simulink model "FFR_3area_4"  (R2015a)
settings: Solver=ode45  StartTime=0.0  StopTime=30  RelTol=1e-3
values from neighbouring files (symbols this model uses):
  beta = [0.3483 0.3827 0.3692]    [init_FFR_3area.m]    (also in init_FFR_3area_2.m; init_FFR_3area_3.m; init_FFR_3area_4.m; init_FFR_3area_5.m)
  D = 0.015    [init_FFR_1_0.m]    (also in init_FFR_1_1.m; init_FFR_3area.m = [0.015 0.016 0.015]; init_FFR_3area_2.m = [0.015 0.016 0.015]; init_FFR_3area_3.m = [0.015 0.016 0.015])
  H = 0.0833    [init_FFR_1_0.m]    (also in init_FFR_1_1.m; init_FFR_3area.m = [0.1667 0.2017 0.1247] .* 0.5; init_FFR_3area_2.m = [0.1667 0.2017 0.1247] .* 0.5; init_FFR_3area_3.m = [0.1667 0.2017 0.1247] .* 0.5)
  Ki = -0.3    [init_FFR_1_0.m]    (also in init_FFR_1_1.m = -2; init_FFR_3area.m = [-0.3 -0.2 -0.4]; init_FFR_3area_2.m = [-0.3 -0.2 -0.4]; init_FFR_3area_3.m = [-0.3 -0.2 -0.4])
  L = 10000    [init_FFR_3area_4.m]    (also in init_FFR_3area_5.m = 1000; init_FRR_3area_6.m = 1000; init_FRR_4area_1.m = 1000)
  MO_down = sortrows(MO_down, 1)    [allocateProduction.m]    (also in allocation.m; init_FFR_3area_4.m; init_FFR_3area_5.m; init_FRR_3area_6.m)
  MO_up = sortrows(MO_up, 1)    [allocateProduction.m]    (also in allocation.m; init_FFR_3area_4.m; init_FFR_3area_5.m; init_FRR_3area_6.m)
  R = 3    [init_FFR_1_0.m]    (also in init_FFR_1_1.m; init_FFR_3area.m = [3 2.73 2.82]; init_FFR_3area_2.m = [3 2.73 2.82]; init_FFR_3area_3.m = [3 2.73 2.82])
  T_12 = 0.20    (= 0.2)    [allocateProduction.m]    (also in allocation.m; init_FFR_3area.m; init_FFR_3area_2.m; init_FFR_3area_3.m)
  T_13 = 0.25    [allocateProduction.m]    (also in allocation.m; init_FFR_3area.m; init_FFR_3area_2.m; init_FFR_3area_3.m)
  T_21 = 0.20    (= 0.2)    [allocateProduction.m]    (also in allocation.m; init_FFR_3area.m; init_FFR_3area_2.m; init_FFR_3area_3.m)
  T_23 = 0.12    [allocateProduction.m]    (also in allocation.m; init_FFR_3area.m; init_FFR_3area_2.m; init_FFR_3area_3.m)
  T_31 = 0.25    [allocateProduction.m]    (also in allocation.m; init_FFR_3area.m; init_FFR_3area_2.m; init_FFR_3area_3.m)
  T_32 = 0.12    [allocateProduction.m]    (also in allocation.m; init_FFR_3area.m; init_FFR_3area_2.m; init_FFR_3area_3.m)
  T_g = 0.08    [init_FFR_1_0.m]    (also in init_FFR_1_1.m; init_FFR_3area.m = [0.08 0.06 0.07]; init_FFR_3area_2.m = [0.08 0.06 0.07]; init_FFR_3area_3.m = [0.08 0.06 0.07])
  T_t = 0.40    (= 0.4)    [init_FFR_1_0.m]    (also in init_FFR_1_1.m; init_FFR_3area.m = [0.40 0.44 0.30]; init_FFR_3area_2.m = [0.40 0.44 0.30]; init_FFR_3area_3.m = [0.40 0.44 0.30])
libraries: simulink x3, aerolibanimutils x1, dspstat3 x1
settings Model: Creator=tarje  LastModifiedBy=tarje

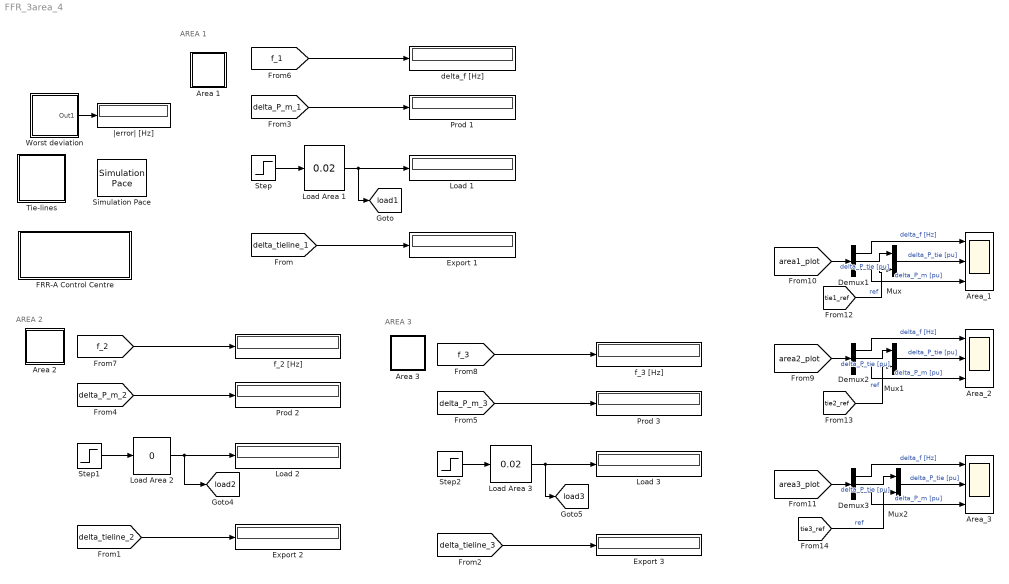
== system FFR_3area_4 ==
  note: AREA 3
  note: AREA 2
  note: AREA 1
  Area 1 : Subsystem
  Area 2 : Subsystem
  Area 3 : Subsystem
  Area_1 : Scope  NumInputPorts=3
      settings: TimeRange=15  YMin=-0.045~-0.015~0.0385  YMax=0.01~0.0175~0.043  SaveName=ScopeData2
  Area_2 : Scope  NumInputPorts=3
      settings: TimeRange=15  YMin=-0.955~-0.2~-0.00045  YMax=-0.855~0.8~0.0007
  Area_3 : Scope  NumInputPorts=3
      settings: TimeRange=15  YMin=-0.965~-0.0575~0.0225  YMax=-0.855~-0.0075~0.0325
  Demux1 : Demux  Outputs=3
  Demux2 : Demux  Outputs=3
  Demux3 : Demux  Outputs=3
  Export 1 : Display
  Export 2 : Display
  Export 3 : Display
  "FRR-A Control Centre " : Subsystem
  Load 1 : Display
  Load 2 : Display
  Load 3 : Display
  Load Area 1 : simulink/Math Operations/Slider Gain  low=-0.2  gain=0.02  high=0.348
  Load Area 2 : simulink/Math Operations/Slider Gain  low=-0.05  gain=0  high=0.348
  Load Area 3 : simulink/Math Operations/Slider Gain  low=-0.05  gain=0.02  high=1
  Mux : Mux  Inputs=2
  Mux1 : Mux  Inputs=2
  Mux2 : Mux  Inputs=2
  Prod 1 : Display
  Prod 2 : Display
  Prod 3 : Display
  Simulation Pace : aerolibanimutils/Simulation Pace  SimulationPace=1  SleepMode=MATLAB Thread  OutputPaceError=off  SampleTime=1/30
      settings: AttributesFormatString=%<SimulationPace> sec/sec
  Step : Step  Time=2  SampleTime=0
  Step1 : Step  Time=2  SampleTime=0
  Step2 : Step  Time=2  SampleTime=0
  Tie-lines : Subsystem
  Worst deviation : Subsystem
  delta_f [Hz] : Display
  f_2 [Hz] : Display
  f_3 [Hz] : Display
  |error| [Hz] : Display
  tag scope: load1=global, load2=global, load3=global
  wires:
  [f_1] -> delta_f [Hz]/1
  [delta_P_m_1] -> Prod 1/1
  Step/1 -> Load Area 1/1
  Load Area 1/1 -> [load1], Load 1/1
  [f_2] -> f_2 [Hz]/1
  [delta_P_m_2] -> Prod 2/1
  Step1/1 -> Load Area 2/1
  Load Area 2/1 -> [load2], Load 2/1
  [f_3] -> f_3 [Hz]/1
  [delta_P_m_3] -> Prod 3/1
  Step2/1 -> Load Area 3/1
  Load Area 3/1 -> [load3], Load 3/1
  [delta_tieline_1] -> Export 1/1
  [delta_tieline_2] -> Export 2/1
  [delta_tieline_3] -> Export 3/1
  Worst deviation/1(Out1) -> |error| [Hz]/1
  [area1_plot] -> Demux1/1
  Demux1/1 -> Area_1/1  "delta_f [Hz]"
  Demux1/2 -> Mux/1  "delta_P_tie [pu]"
  Demux1/3 -> Area_1/3  "delta_P_m [pu]"
  [area2_plot] -> Demux2/1
  Demux2/1 -> Area_2/1  "delta_f [Hz]"
  Demux2/2 -> Mux1/1  "delta_P_tie [pu]"
  Demux2/3 -> Area_2/3  "delta_P_m [pu]"
  [area3_plot] -> Demux3/1
  Demux3/1 -> Area_3/1  "delta_f [Hz]"
  Demux3/2 -> Mux2/1  "delta_P_tie [pu]"
  Demux3/3 -> Area_3/3  "delta_P_m [pu]"
  Mux/1 -> Area_1/2  "delta_P_tie [pu]"
  [tie1_ref] -> Mux/2  "ref"
  [tie2_ref] -> Mux1/2  "ref"
  Mux1/1 -> Area_2/2  "delta_P_tie [pu]"
  Mux2/1 -> Area_3/2  "delta_P_tie [pu]"
  [tie3_ref] -> Mux2/2  "ref"

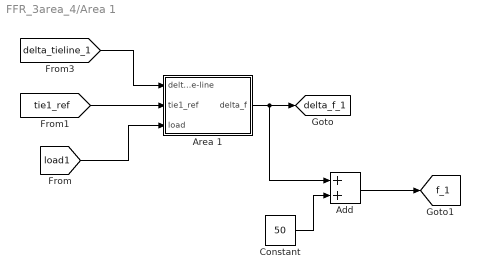
== system FFR_3area_4/Area 1 ==
  Add : Sum
  Area 1 : Subsystem
  Constant : Constant  Value=50
  tag scope: delta_f_1=global, f_1=global
  wires:
  [delta_tieline_1] -> Area 1/1(delta_tie-line)
  Area 1/1(delta_f) -> Add/1, [delta_f_1]
  [load1] -> Area 1/3(load)
  Constant/1 -> Add/2
  Add/1 -> [f_1]
  [tie1_ref] -> Area 1/2(tie1_ref)

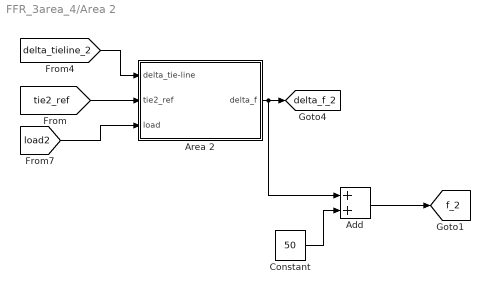
== system FFR_3area_4/Area 2 ==
  Add : Sum
  Area 2 : Subsystem
  Constant : Constant  Value=50
  tag scope: delta_f_2=global, f_2=global
  wires:
  Area 2/1(delta_f) -> Add/1, [delta_f_2]
  [load2] -> Area 2/3(load)
  [delta_tieline_2] -> Area 2/1(delta_tie-line)
  Constant/1 -> Add/2
  Add/1 -> [f_2]
  [tie2_ref] -> Area 2/2(tie2_ref)

== system FFR_3area_4/Area 3 ==
  Add : Sum
  Area 3 : Subsystem
  Constant2 : Constant  Value=50
  tag scope: delta_f_3=global, f_3=global
  wires:
  [load3] -> Area 3/3(load)
  Area 3/1(delta_f) -> Add/1, [delta_f_3]
  [delta_tieline_3] -> Area 3/1(delta_tie-line)
  Add/1 -> [f_3]
  Constant2/1 -> Add/2
  [tie3_ref] -> Area 3/2(tie3_ref)

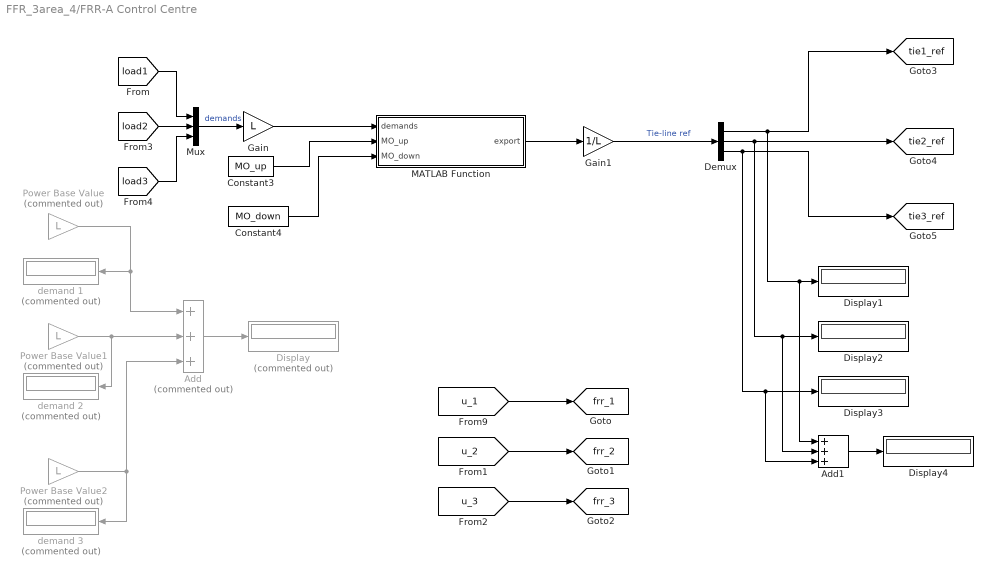
== system FFR_3area_4/FRR-A Control Centre  ==
  Add : Sum  Commented=on  Inputs=+++
  Add1 : Sum  Inputs=3
  Constant3 : Constant  Value=MO_up
  Constant4 : Constant  Value=MO_down
  Demux : Demux  Outputs=3
  Display : Display  Commented=on
  Display{1..4} (4 alike) : Display
  Gain : Gain  Gain=L
  Gain1 : Gain  Gain=1/L
  MATLAB Function : MATLAB Function  TreatAsAtomicUnit=on  SystemSampleTime=2
  Mux : Mux  Inputs=3
  Power Base Value : Gain  Commented=on  Gain=L
  Power Base Value1 : Gain  Commented=on  Gain=L
  Power Base Value2 : Gain  Commented=on  Gain=L
  demand 1 : Display  Commented=on
  demand 2 : Display  Commented=on
  demand 3 : Display  Commented=on
  tag scope: frr_1=global, frr_2=global, frr_3=global, tie1_ref=global, tie2_ref=global, tie3_ref=global
  wires:
  Add/1 -> Display/1
  Power Base Value/1 -> demand 1/1, Add/1
  Power Base Value1/1 -> demand 2/1, Add/2
  Power Base Value2/1 -> demand 3/1, Add/3
  [u_1] -> [frr_1]
  [u_2] -> [frr_2]
  [u_3] -> [frr_3]
  [load2] -> Mux/2
  [load1] -> Mux/1
  [load3] -> Mux/3
  Mux/1 -> Gain/1  "demands"
  Gain1/1 -> Demux/1  "Tie-line ref"
  Constant3/1 -> MATLAB Function/2(MO_up)
  Constant4/1 -> MATLAB Function/3(MO_down)
  Gain/1 -> MATLAB Function/1(demands)
  MATLAB Function/1(export) -> Gain1/1
  Demux/1 -> Add1/1, Display1/1, [tie1_ref]
  Demux/2 -> Add1/2, Display2/1, [tie2_ref]
  Demux/3 -> Add1/3, Display3/1, [tie3_ref]
  Add1/1 -> Display4/1

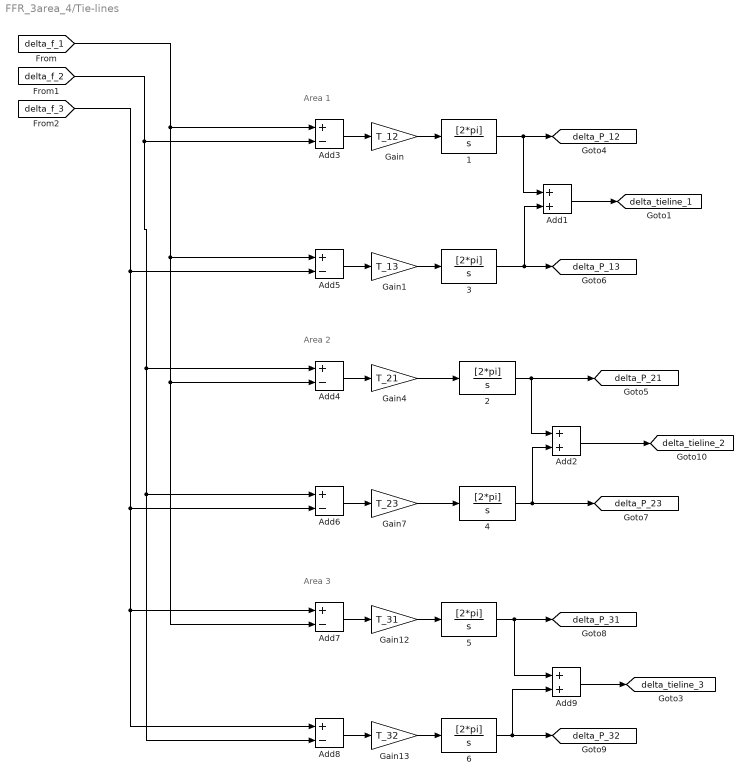
== system FFR_3area_4/Tie-lines ==
  note: Area 3
  note: Area 2
  note: Area 1
   {1..6} (6 alike) : TransferFcn  Numerator=[2*pi]  Denominator=[1 0]
  Add1 : Sum
  Add2 : Sum
  Add{3..8} (6 alike) : Sum  Inputs=+-
  Add9 : Sum
  Gain : Gain  Gain=T_12
  Gain1 : Gain  Gain=T_13
  Gain12 : Gain  Gain=T_31
  Gain13 : Gain  Gain=T_32
  Gain4 : Gain  Gain=T_21
  Gain7 : Gain  Gain=T_23
  tag scope: delta_P_12=global, delta_P_13=global, delta_P_21=global, delta_P_23=global, delta_P_31=global, delta_P_32=global, delta_tieline_1=global, delta_tieline_2=global, delta_tieline_3=global
  wires:
  [delta_f_2] -> Add3/2, Add8/2, Add6/1, Add4/1
  [delta_f_1] -> Add3/1, Add5/1, Add7/2, Add4/2
  [delta_f_3] -> Add5/2, Add8/1, Add7/1, Add6/2
  " 1"/1 -> Add1/1, [delta_P_12]
  Add3/1 -> Gain/1
  " 2"/1 -> Add2/1, [delta_P_21]
  Add4/1 -> Gain4/1
  " 3"/1 -> Add1/2, [delta_P_13]
  Add5/1 -> Gain1/1
  " 4"/1 -> Add2/2, [delta_P_23]
  Add6/1 -> Gain7/1
  " 5"/1 -> Add9/1, [delta_P_31]
  Add7/1 -> Gain12/1
  " 6"/1 -> Add9/2, [delta_P_32]
  Add8/1 -> Gain13/1
  Add9/1 -> [delta_tieline_3]
  Gain12/1 -> " 5"/1
  Gain13/1 -> " 6"/1
  Add2/1 -> [delta_tieline_2]
  Gain4/1 -> " 2"/1
  Gain7/1 -> " 4"/1
  Add1/1 -> [delta_tieline_1]
  Gain/1 -> " 1"/1
  Gain1/1 -> " 3"/1

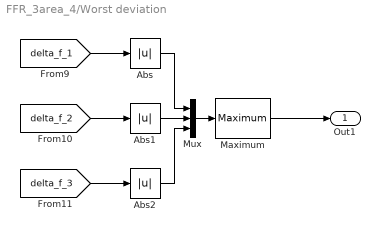
== system FFR_3area_4/Worst deviation ==
  Abs : Abs
  Abs1 : Abs
  Abs2 : Abs
  Maximum : dspstat3/Maximum  fcn=Value  reset=None  InputProcessing=Columns as channels (frame based)  indexBase=One  operateOver=Each column  Dimension=1  colComp=on  operation=maximum  roiEnable=off  roiType=Rectangles  roiPortion=Entire ROI  roiOutput=Individual statistics for each ROI  roiFlag=off  accumDataTypeStr=Inherit: Same as product output  accumLastDataTypeStr=Inherit: Same as product output  roundingMode=Ceiling  overflowMode=off
  Mux : Mux  Inputs=3
  Out1 : Outport
  wires:
  Maximum/1 -> Out1/1
  Abs2/1 -> Mux/3
  Mux/1 -> Maximum/1
  [delta_f_2] -> Abs1/1
  [delta_f_3] -> Abs2/1
  Abs/1 -> Mux/1
  Abs1/1 -> Mux/2
  [delta_f_1] -> Abs/1

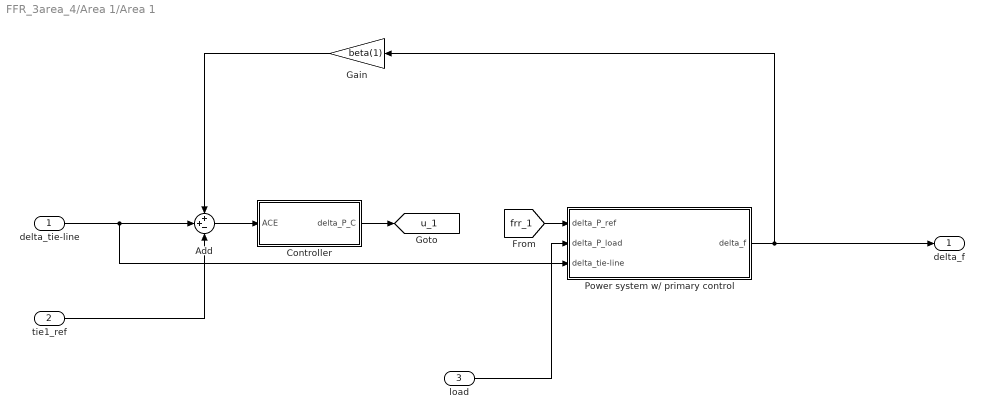
== system FFR_3area_4/Area 1/Area 1 ==
  delta_tie-line : Inport
  tie1_ref : Inport  Port=2
  load : Inport  Port=3
  Add : Sum  Inputs=++-
  Controller : Subsystem
  Gain : Gain  Gain=beta(1)
  Power system w/ primary control : Subsystem
  delta_f : Outport
  tag scope: u_1=global
  wires:
  Power system w/ primary control/1(delta_f) -> Gain/1, delta_f/1
  Gain/1 -> Add/1
  delta_tie-line/1 -> Power system w/ primary control/3(delta_tie-line), Add/2
  load/1 -> Power system w/ primary control/2(delta_P_load)
  [frr_1] -> Power system w/ primary control/1(delta_P_ref)
  Controller/1(delta_P_C) -> [u_1]
  Add/1 -> Controller/1(ACE)
  tie1_ref/1 -> Add/3

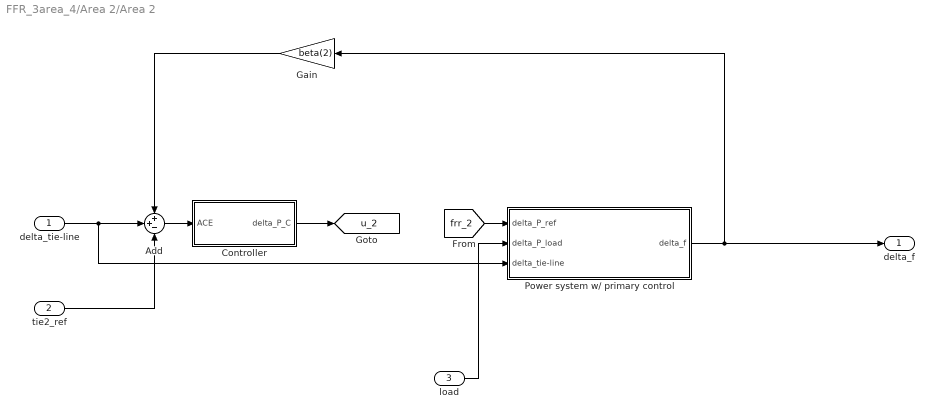
== system FFR_3area_4/Area 2/Area 2 ==
  delta_tie-line : Inport
  tie2_ref : Inport  Port=2
  load : Inport  Port=3
  Add : Sum  Inputs=++-
  Controller : Subsystem
  Gain : Gain  Gain=beta(2)
  Power system w/ primary control : Subsystem
  delta_f : Outport
  tag scope: u_2=global
  wires:
  Power system w/ primary control/1(delta_f) -> Gain/1, delta_f/1
  Gain/1 -> Add/1
  delta_tie-line/1 -> Power system w/ primary control/3(delta_tie-line), Add/2
  Add/1 -> Controller/1(ACE)
  load/1 -> Power system w/ primary control/2(delta_P_load)
  [frr_2] -> Power system w/ primary control/1(delta_P_ref)
  Controller/1(delta_P_C) -> [u_2]
  tie2_ref/1 -> Add/3

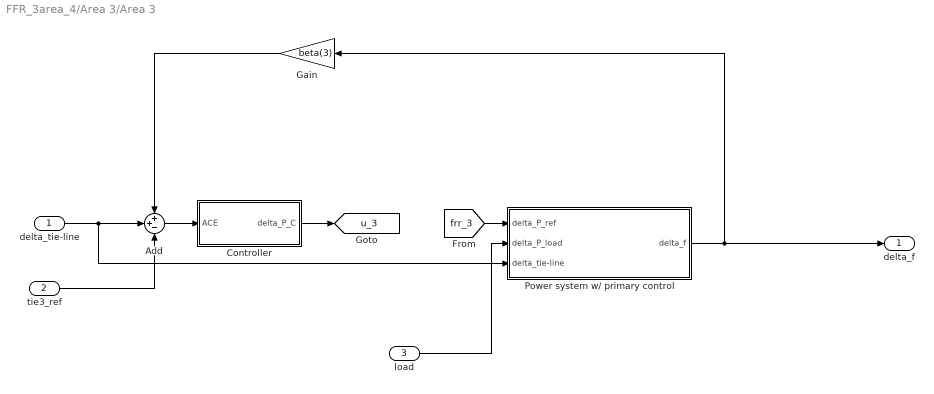
== system FFR_3area_4/Area 3/Area 3 ==
  delta_tie-line : Inport
  tie3_ref : Inport  Port=2
  load : Inport  Port=3
  Add : Sum  Inputs=++-
  Controller : Subsystem
  Gain : Gain  Gain=beta(3)
  Power system w/ primary control : Subsystem
  delta_f : Outport
  tag scope: u_3=global
  wires:
  Power system w/ primary control/1(delta_f) -> Gain/1, delta_f/1
  Gain/1 -> Add/1
  delta_tie-line/1 -> Power system w/ primary control/3(delta_tie-line), Add/2
  Add/1 -> Controller/1(ACE)
  load/1 -> Power system w/ primary control/2(delta_P_load)
  [frr_3] -> Power system w/ primary control/1(delta_P_ref)
  Controller/1(delta_P_C) -> [u_3]
  tie3_ref/1 -> Add/3

== system FFR_3area_4/Area 1/Area 1/Controller ==
  ACE : Inport
  Transfer Fcn : TransferFcn  Numerator=[Ki(1)]  Denominator=[1 0]
  delta_P_C : Outport
  wires:
  ACE/1 -> Transfer Fcn/1
  Transfer Fcn/1 -> delta_P_C/1

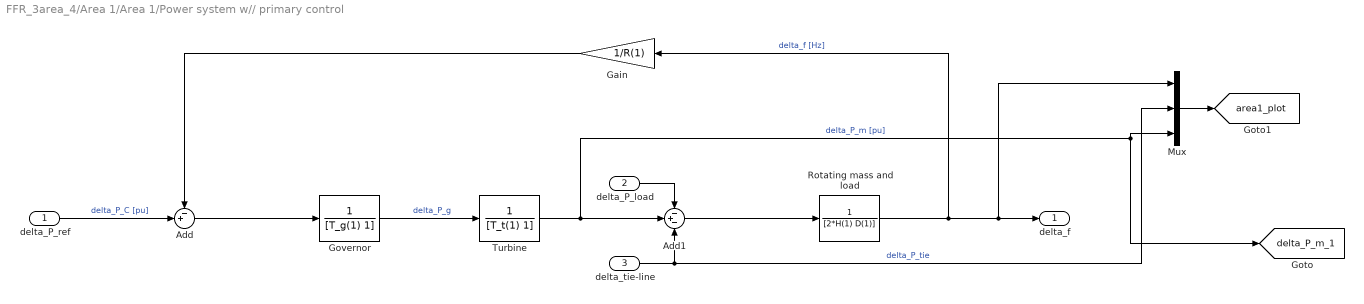
== system FFR_3area_4/Area 1/Area 1/Power system w// primary control ==
  delta_P_ref : Inport
  delta_P_load : Inport  Port=2
  delta_tie-line : Inport  Port=3
  Add : Sum  Inputs=-+|
  Add1 : Sum  Inputs=-+-
  Gain : Gain  Gain=1/R(1)
  Governor : TransferFcn  Denominator=[T_g(1) 1]
  Mux : Mux  Inputs=3
  Rotating mass and load : TransferFcn  Denominator=[2*H(1) D(1)]
  Turbine : TransferFcn  Denominator=[T_t(1) 1]
  delta_f : Outport
  tag scope: area1_plot=global, delta_P_m_1=global
  wires:
  Turbine/1 -> Mux/3, [delta_P_m_1], Add1/2  "delta_P_m [pu]"
  Rotating mass and load/1 -> Mux/1, delta_f/1, Gain/1  "delta_f [Hz]"
  Gain/1 -> Add/1
  Add1/1 -> Rotating mass and load/1
  Add/1 -> Governor/1
  Governor/1 -> Turbine/1  "delta_P_g"
  delta_P_ref/1 -> Add/2  "delta_P_C [pu]"
  delta_P_load/1 -> Add1/1
  delta_tie-line/1 -> Mux/2, Add1/3  "delta_P_tie"
  Mux/1 -> [area1_plot]

== system FFR_3area_4/Area 2/Area 2/Controller ==
  ACE : Inport
  Transfer Fcn : TransferFcn  Numerator=[Ki(2)]  Denominator=[1 0]
  delta_P_C : Outport
  wires:
  ACE/1 -> Transfer Fcn/1
  Transfer Fcn/1 -> delta_P_C/1

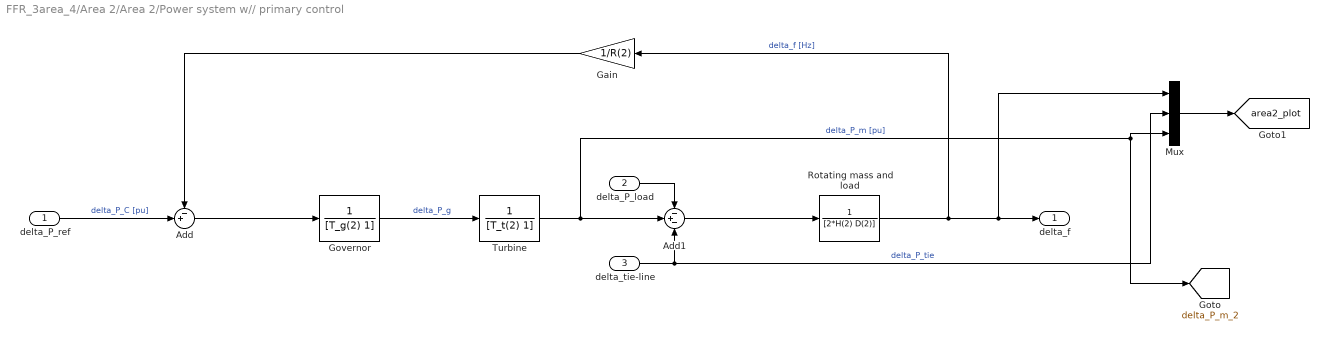
== system FFR_3area_4/Area 2/Area 2/Power system w// primary control ==
  delta_P_ref : Inport
  delta_P_load : Inport  Port=2
  delta_tie-line : Inport  Port=3
  Add : Sum  Inputs=-+|
  Add1 : Sum  Inputs=-+-
  Gain : Gain  Gain=1/R(2)
  Governor : TransferFcn  Denominator=[T_g(2) 1]
  Mux : Mux  Inputs=3
  Rotating mass and load : TransferFcn  Denominator=[2*H(2) D(2)]
  Turbine : TransferFcn  Denominator=[T_t(2) 1]
  delta_f : Outport
  tag scope: area2_plot=global, delta_P_m_2=global
  wires:
  Turbine/1 -> Mux/3, [delta_P_m_2], Add1/2  "delta_P_m [pu]"
  Rotating mass and load/1 -> Mux/1, delta_f/1, Gain/1  "delta_f [Hz]"
  Gain/1 -> Add/1
  Add1/1 -> Rotating mass and load/1
  Add/1 -> Governor/1
  Governor/1 -> Turbine/1  "delta_P_g"
  delta_P_ref/1 -> Add/2  "delta_P_C [pu]"
  delta_P_load/1 -> Add1/1
  delta_tie-line/1 -> Mux/2, Add1/3  "delta_P_tie"
  Mux/1 -> [area2_plot]

== system FFR_3area_4/Area 3/Area 3/Controller ==
  ACE : Inport
  Transfer Fcn : TransferFcn  Numerator=[Ki(3)]  Denominator=[1 0]
  delta_P_C : Outport
  wires:
  ACE/1 -> Transfer Fcn/1
  Transfer Fcn/1 -> delta_P_C/1

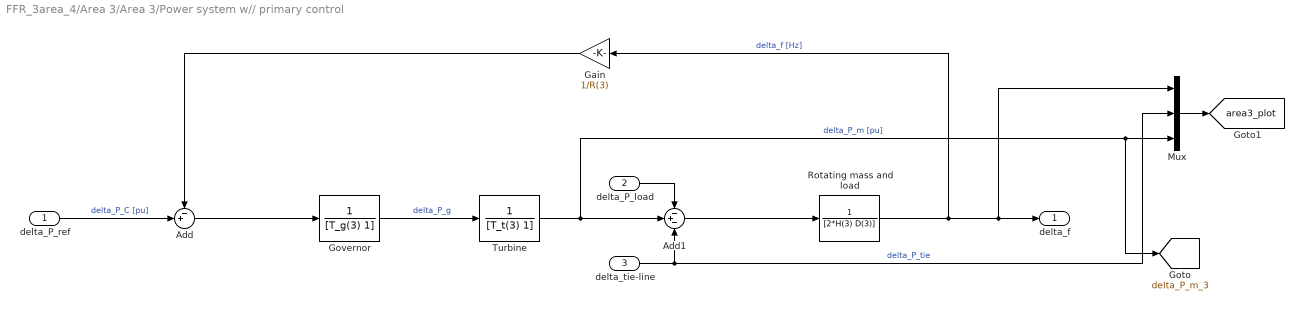
== system FFR_3area_4/Area 3/Area 3/Power system w// primary control ==
  delta_P_ref : Inport
  delta_P_load : Inport  Port=2
  delta_tie-line : Inport  Port=3
  Add : Sum  Inputs=-+|
  Add1 : Sum  Inputs=-+-
  Gain : Gain  Gain=1/R(3)
  Governor : TransferFcn  Denominator=[T_g(3) 1]
  Mux : Mux  Inputs=3
  Rotating mass and load : TransferFcn  Denominator=[2*H(3) D(3)]
  Turbine : TransferFcn  Denominator=[T_t(3) 1]
  delta_f : Outport
  tag scope: area3_plot=global, delta_P_m_3=global
  wires:
  Turbine/1 -> [delta_P_m_3], Mux/3, Add1/2  "delta_P_m [pu]"
  Rotating mass and load/1 -> Mux/1, delta_f/1, Gain/1  "delta_f [Hz]"
  Gain/1 -> Add/1
  Add1/1 -> Rotating mass and load/1
  Add/1 -> Governor/1
  Governor/1 -> Turbine/1  "delta_P_g"
  delta_P_ref/1 -> Add/2  "delta_P_C [pu]"
  delta_P_load/1 -> Add1/1
  delta_tie-line/1 -> Mux/2, Add1/3  "delta_P_tie"
  Mux/1 -> [area3_plot]

== matlab function FFR_3area_4/FRR-A Control Centre /MATLAB Function ==
  data: demands input; export output; MO_up input; MO_down input
function export = fcn(demands, MO_up, MO_down)

% Define variables
PRICE = 1;
QUANTITY = 2;
AREA = 3;
LEFT = 4;

prod = zeros(length(demands),1);

% Sum demands
demand = sum(demands);

% If frequency is too low
if demand >= 0
    % Check if MO_up is empty
    for i = 1:length(MO_up)
        q = MO_up(i, QUANTITY);
        if demand > q
            prod(MO_up(i,AREA)) = prod(MO_up(i,AREA)) + q;
            demand = demand - q;
        else
             prod(MO_up(i,AREA)) = prod(MO_up(i,AREA)) + demand;
             demand = 0;
             break;
        end
    end
    if demand ~= 0
        % Not enough UP-bids
    end
% If frequency is too high
else
    demand = abs(demand); % Change sign of demand
    % Check if MO_down is empty
    for i = 1:length(MO_down)
        q = MO_down(i, QUANTITY);
        if demand > q
            prod(MO_down(i,AREA)) = prod(MO_down(i,AREA)) - q;
            demand = demand - q;
        else
             prod(MO_down(i,AREA)) = prod(MO_down(i,AREA)) - demand;
             demand = 0;
             break;
        end
    end
    if demand ~= 0
        % Not enough DOWN-bids
    end
end

% Solve bill settle problem
export = prod - sum(prod)/length(prod);


end
